simulink model "hydraulic"  (R2015b)
settings: Solver=ode23t  StartTime=0.0  StopTime=5  RelTol=1e-3
values from neighbouring files (symbols this model uses):
  A = [zeros(2) eye(2);-[kf/J1 -kf/J1;-kf/J2 kf/J2] -[df/J1 -df/J1;-df/J2 df/J2]]    [ex5.m]    (also in ex6.m = [-df/m Am/m -Am/m)
  A1 = Am    (= 0.00180641577581)    [ex6.m]
  A2 = Am    (= 0.00180641577581)    [ex6.m]
  B = [0 0 J_m/J1 0]'    [ex5.m]    (also in ex6.m = [ 0 -1/m)
  C = [0 0 1 0]    [ex5.m]    (also in ex6.m = [1 0 0; 0 1 0; 0 0 1])
  Cf = V0/B    (= 6.87223392973e-13)    [ex6.m]
  D = [0; 0]    [ex1.m]    (also in ex6.m = [0 0; 0 0; 0 0])
  df = 0.0001    [ex5.m]    (also in ex6.m = 200)
  Fe = 10000    [ex6.m]
  m = 100    [ex6.m]
  p10 = double(solution.p1)    [ex6.m]
  p20 = double(solution.p2)    [ex6.m]
  Ps = 20e6    (= 20000000)    [ex6.m]
  Rv = 1e-4    (= 0.0001)    [ex6.m]
  Tforce = 1    [ex6.m]
  xv = 0.01    [ex6.m]
settings Model: Creator=gabri  LastModifiedBy=Gabriel

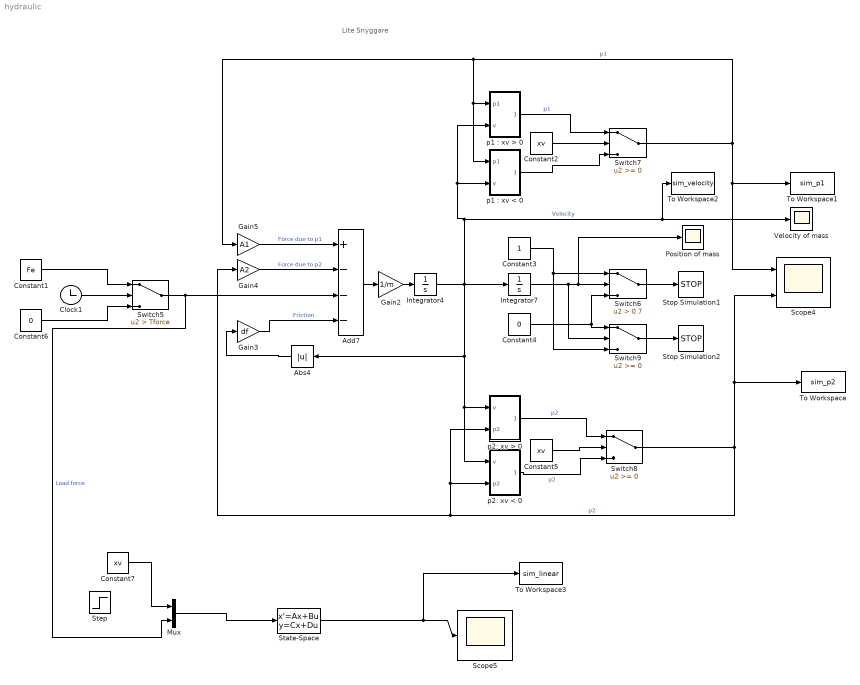
== system hydraulic ==
  note: Lite Snyggare
  Abs4 : Abs
  Add7 : Sum  Inputs=+---
  Clock1 : Clock
  Constant1 : Constant  Value=Fe
  Constant2 : Constant  Value=xv
  Constant3 : Constant
  Constant4 : Constant  Value=0
  Constant5 : Constant  Value=xv
  Constant6 : Constant  Value=0
  Constant7 : Constant  Value=xv
  Gain2 : Gain  Gain=1/m
  Gain3 : Gain  Gain=df
  Gain4 : Gain  Gain=A2
  Gain5 : Gain  Gain=A1
  Integrator4 : Integrator
  Integrator7 : Integrator
  Mux : Mux  Inputs=2
  Position of mass : Scope
  Scope4 : Scope  NumInputPorts=2
  Scope5 : Scope
  State-Space : StateSpace  A=A  B=B  C=C  D=D  X0=0
  Step : Step  Time=0  After=0.01  SampleTime=0
  Stop Simulation1 : Stop
  Stop Simulation2 : Stop
  Switch5 : Switch  Criteria=u2 > Threshold  Threshold=Tforce
  Switch6 : Switch  Criteria=u2 > Threshold  Threshold=0.7
  Switch7 : Switch
  Switch8 : Switch
  Switch9 : Switch
  To Workspace : ToWorkspace  VariableName=sim_p2  SaveFormat=Timeseries  SampleTime=-1
  To Workspace1 : ToWorkspace  VariableName=sim_p1  SaveFormat=Timeseries  SampleTime=-1
  To Workspace2 : ToWorkspace  VariableName=sim_velocity  SaveFormat=Timeseries  SampleTime=-1
  To Workspace3 : ToWorkspace  VariableName=sim_linear  SaveFormat=Timeseries  SampleTime=-1
  Velocity of mass : Scope
  "p1 : xv < 0" : Subsystem
  "p1 : xv > 0" : Subsystem
  p2: xv < 0 : Subsystem
  "p2: xv > 0 " : Subsystem
  wires:
  Clock1/1 -> Switch5/2
  Constant1/1 -> Switch5/1
  Gain4/1 -> Add7/2  "Force due to p2"
  Add7/1 -> Gain2/1
  Gain2/1 -> Integrator4/1
  Integrator4/1 -> Integrator7/1, "p1 : xv < 0"/2(v), "p1 : xv > 0"/2(v), To Workspace2/1, Velocity of mass/1, Abs4/1, "p2: xv > 0 "/1(v), p2: xv < 0/1(v)  "Velocity"
  Switch6/1 -> Stop Simulation1/1
  Constant3/1 -> Switch9/3, Switch6/1
  Constant4/1 -> Switch6/3, Switch9/1
  "p1 : xv > 0"/1(Out1) -> Switch7/1  "p1"
  "p1 : xv < 0"/1(Out1) -> Switch7/3
  Constant2/1 -> Switch7/2
  Switch7/1 -> "p1 : xv > 0"/1("p1 "), "p1 : xv < 0"/1(p1), Gain5/1, Scope4/1, To Workspace1/1  "p1"
  Constant5/1 -> Switch8/2
  Switch8/1 -> p2: xv < 0/2(p2), "p2: xv > 0 "/2(p2), Gain4/1, Scope4/2, To Workspace/1  "p2"
  p2: xv < 0/1(Out1) -> Switch8/3  "p2"
  "p2: xv > 0 "/1(Out1) -> Switch8/1  "p2"
  Gain3/1 -> Add7/4  "Friction"
  Integrator7/1 -> Switch9/2, Position of mass/1, Switch6/2
  Gain5/1 -> Add7/1  "Force due to p1"
  Switch9/1 -> Stop Simulation2/1
  Abs4/1 -> Gain3/1
  Constant6/1 -> Switch5/3
  Switch5/1 -> Mux/2, Add7/3  "Load force"
  State-Space/1 -> To Workspace3/1, Scope5/1
  Mux/1 -> State-Space/1
  Constant7/1 -> Mux/1

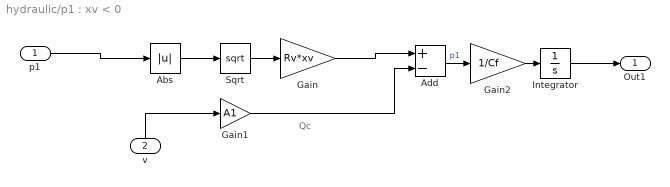
== system hydraulic/p1 : xv < 0 ==
  note: Qc
  p1 : Inport
  v : Inport  Port=2
  Abs : Abs
  Add : Sum  Inputs=+-
  Gain : Gain  Gain=Rv*xv
  Gain1 : Gain  Gain=A1
  Gain2 : Gain  Gain=1/Cf
  Integrator : Integrator
  Sqrt : Sqrt  SaturateOnIntegerOverflow=on
  Out1 : Outport
  wires:
  v/1 -> Gain1/1
  Gain1/1 -> Add/2
  Abs/1 -> Sqrt/1
  p1/1 -> Abs/1
  Add/1 -> Gain2/1  "p1"
  Gain2/1 -> Integrator/1
  Integrator/1 -> Out1/1
  Sqrt/1 -> Gain/1
  Gain/1 -> Add/1

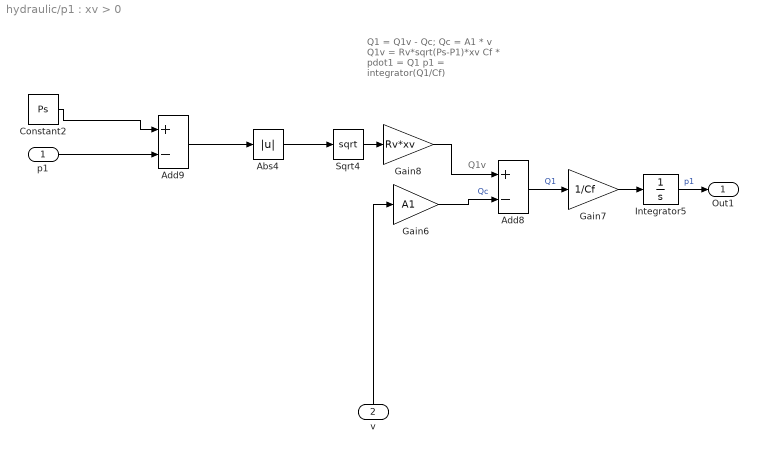
== system hydraulic/p1 : xv > 0 ==
  note: Q1v
  note: Q1 = Q1v - Qc;
      | Qc = A1 * v
      | Q1v = Rv*sqrt(Ps-P1)*xv
      | Cf * pdot1 = Q1
      | p1 = integrator(Q1/Cf)
  "p1 " : Inport
  v : Inport  Port=2
  Abs4 : Abs
  Add8 : Sum  Inputs=+-
  Add9 : Sum  Inputs=+-
  Constant2 : Constant  Value=Ps
  Gain6 : Gain  Gain=A1
  Gain7 : Gain  Gain=1/Cf
  Gain8 : Gain  Gain=Rv*xv
  Integrator5 : Integrator  InitialCondition=p10
  Sqrt4 : Sqrt  SaturateOnIntegerOverflow=on
  Out1 : Outport
  wires:
  Add9/1 -> Abs4/1
  Constant2/1 -> Add9/1
  Abs4/1 -> Sqrt4/1
  Gain7/1 -> Integrator5/1
  Gain6/1 -> Add8/2  "Qc"
  Integrator5/1 -> Out1/1  "p1"
  Add8/1 -> Gain7/1  "Q1"
  Sqrt4/1 -> Gain8/1
  Gain8/1 -> Add8/1
  v/1 -> Gain6/1
  "p1 "/1 -> Add9/2

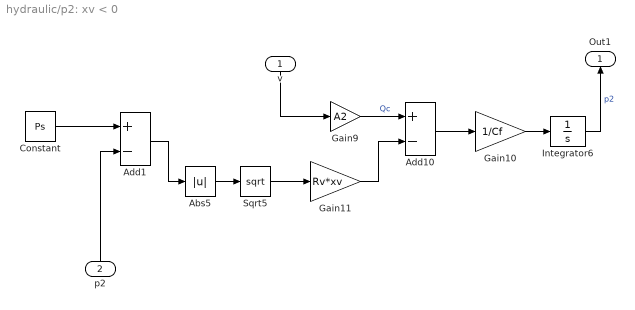
== system hydraulic/p2: xv < 0 ==
  v : Inport
  p2 : Inport  Port=2
  Abs5 : Abs
  Add1 : Sum  Inputs=+-
  Add10 : Sum  Inputs=+-
  Constant : Constant  Value=Ps
  Gain10 : Gain  Gain=1/Cf
  Gain11 : Gain  Gain=Rv*xv
  Gain9 : Gain  Gain=A2
  Integrator6 : Integrator
  Sqrt5 : Sqrt  SaturateOnIntegerOverflow=on
  Out1 : Outport
  wires:
  Abs5/1 -> Sqrt5/1
  Gain9/1 -> Add10/1  "Qc"
  Sqrt5/1 -> Gain11/1
  Gain10/1 -> Integrator6/1
  Add10/1 -> Gain10/1
  Integrator6/1 -> Out1/1  "p2"
  v/1 -> Gain9/1
  p2/1 -> Add1/2
  Add1/1 -> Abs5/1
  Constant/1 -> Add1/1
  Gain11/1 -> Add10/2

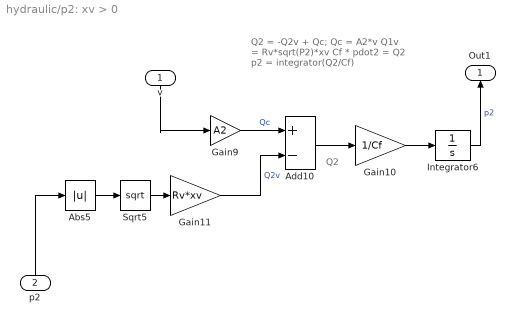
== system hydraulic/p2: xv > 0  ==
  note: Q2
  note: Q2 = -Q2v + Qc;
      | Qc = A2*v
      | Q1v = Rv*sqrt(P2)*xv
      | Cf * pdot2 = Q2
      | p2 = integrator(Q2/Cf)
  v : Inport
  p2 : Inport  Port=2
  Abs5 : Abs
  Add10 : Sum  Inputs=+-
  Gain10 : Gain  Gain=1/Cf
  Gain11 : Gain  Gain=Rv*xv
  Gain9 : Gain  Gain=A2
  Integrator6 : Integrator  InitialCondition=p20
  Sqrt5 : Sqrt  SaturateOnIntegerOverflow=on
  Out1 : Outport
  wires:
  p2/1 -> Abs5/1
  v/1 -> Gain9/1
  Integrator6/1 -> Out1/1  "p2"
  Add10/1 -> Gain10/1
  Gain10/1 -> Integrator6/1
  Sqrt5/1 -> Gain11/1
  Gain11/1 -> Add10/2  "Q2v"
  Gain9/1 -> Add10/1  "Qc"
  Abs5/1 -> Sqrt5/1
